simulink model "Imu_sensor_module"  (R2024b)
settings: Solver=VariableStepAuto  StartTime=0.0  StopTime=10  RelTol=1e-3
values from neighbouring files (symbols this model uses):
  bias_acc = [0.01; -0.02; 0.005]    [CalibParams.m]    (also in Calibrated_Data.mat = [-0.00255529989353 0.0383310681174 -0.0164973505603]; ImuCalibrationGui.m = app.BiasAcc)
  bias_gyro = [0.005; -0.005; 0.002]    [CalibParams.m]    (also in Calibrated_Data.mat = [-0.411069831507 0.447881147736 1.44802201926]; ImuCalibrationGui.m = app.BiasGyro)
  scale_acc = [1.01; 0.98; 1.03]    [CalibParams.m]    (also in Calibrated_Data.mat = [2.19824309405 1.51064702678 3.24094019827]; ImuCalibrationGui.m = app.ScaleAcc)
  scale_gyro = [1.00; 1.02; 0.99]    [CalibParams.m]    (also in Calibrated_Data.mat = [1.88477128946 2.18055047165 4.18647933973]; ImuCalibrationGui.m = app.ScaleGyro)
libraries: simulink x6, sharedtransform x1
settings Model: Creator=Admin  LastModifiedBy=Admin
settings DataIOCC: SaveOutput=off  SignalLogging=off  ReturnWorkspaceOutputs=off

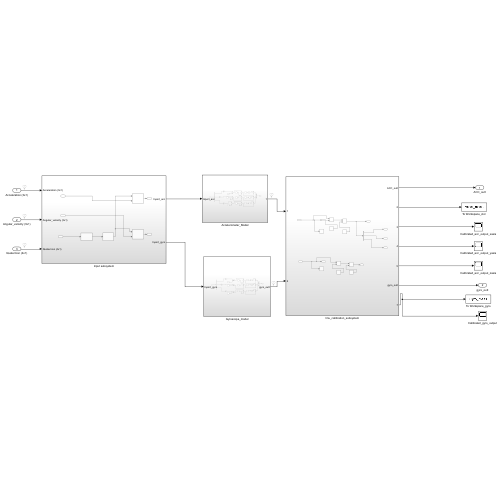
[thumbnail: Simulink's stored preview of the top-level diagram]
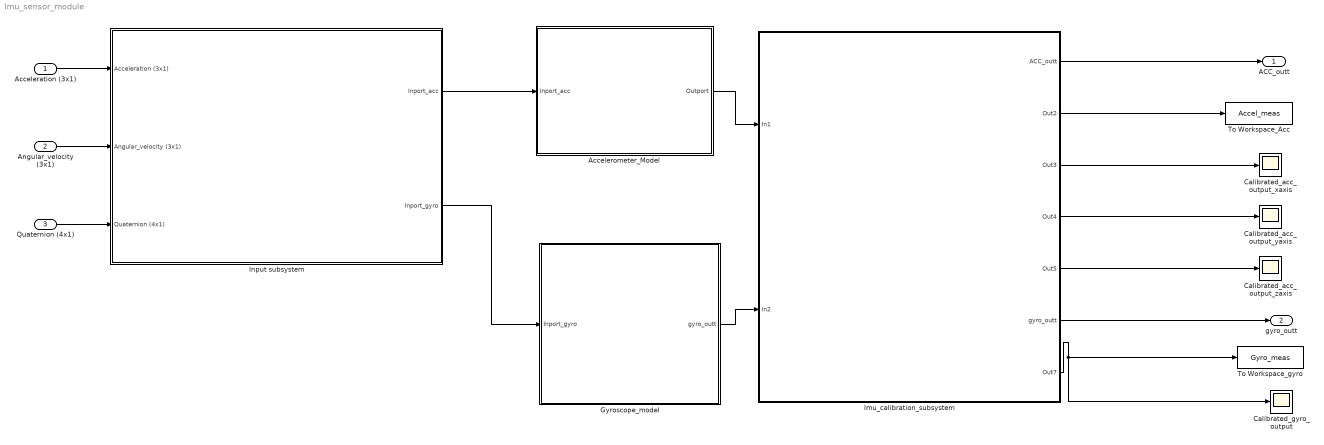
== system Imu_sensor_module ==
  Acceleration (3x1) : Inport  PortDimensions=[3 1]
  Angular_velocity (3x1) : Inport  Port=2  PortDimensions=[3 1]
  Quaternion (4x1) : Inport  Port=3  PortDimensions=[4 1]
  Accelerometer_Model : Subsystem
  Calibrated_acc_output_xaxis : Scope
  Calibrated_acc_output_yaxis : Scope
  Calibrated_acc_output_zaxis : Scope
  Calibrated_gyro_output : Scope
  Gyroscope_model : Subsystem
  Imu_calibration_subsystem : Subsystem
  Input subsystem : Subsystem
  To Workspace_Acc : ToWorkspace  VariableName=Accel_meas  SaveFormat=Structure With Time  SampleTime=-1
  To Workspace_gyro : ToWorkspace  VariableName=Gyro_meas  SaveFormat=Structure With Time  SampleTime=-1
  ACC_outt : Outport
  gyro_outt : Outport  Port=2
  wires:
  Acceleration (3x1)/1 -> Input subsystem/1(Acceleration (3x1))
  Angular_velocity (3x1)/1 -> Input subsystem/2(Angular_velocity (3x1))
  Quaternion (4x1)/1 -> Input subsystem/3(Quaternion (4x1))
  Input subsystem/1(Inport_acc) -> Accelerometer_Model/1(Inport_acc)
  Input subsystem/2(Inport_gyro) -> Gyroscope_model/1(Inport_gyro)
  Imu_calibration_subsystem/7(Out7) -> To Workspace_gyro/1, Calibrated_gyro_output/1
  Accelerometer_Model/1(Outport) -> Imu_calibration_subsystem/1(In1)
  Gyroscope_model/1(gyro_outt) -> Imu_calibration_subsystem/2(In2)
  Imu_calibration_subsystem/1(ACC_outt) -> ACC_outt/1
  Imu_calibration_subsystem/2(Out2) -> To Workspace_Acc/1
  Imu_calibration_subsystem/3(Out3) -> Calibrated_acc_output_xaxis/1
  Imu_calibration_subsystem/4(Out4) -> Calibrated_acc_output_yaxis/1
  Imu_calibration_subsystem/5(Out5) -> Calibrated_acc_output_zaxis/1
  Imu_calibration_subsystem/6(gyro_outt) -> gyro_outt/1

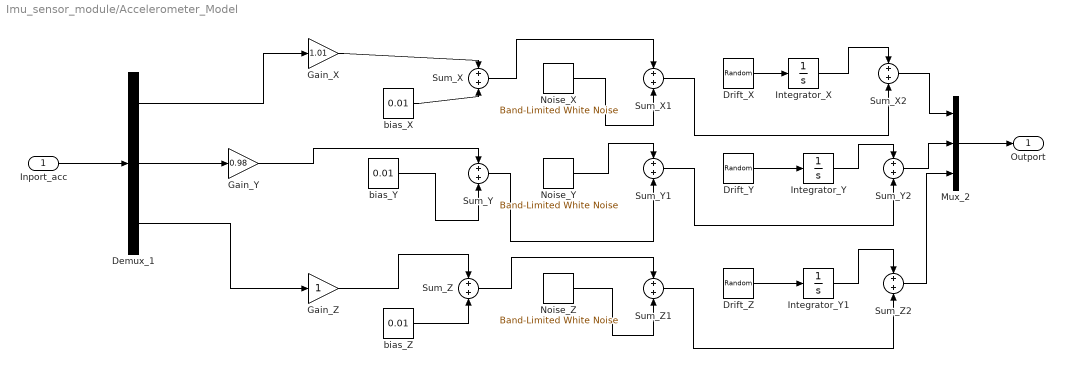
== system Imu_sensor_module/Accelerometer_Model ==
  Inport_acc : Inport  PortDimensions=[3 1]
  Demux_1 : Demux  Outputs=3
  "Drift_X " : RandomNumber  Variance=9e-8  Seed=101  SampleTime=0.01
  Drift_Y : RandomNumber  Variance=7.84e-8  Seed=102  SampleTime=0.01
  Drift_Z : RandomNumber  Variance=6.76e-8  Seed=103  SampleTime=0.01
  Gain_X : Gain  Gain=1.01
  Gain_Y : Gain  Gain=0.98
  Gain_Z : Gain
  "Integrator_X " : Integrator  LimitOutput=on
  Integrator_Y : Integrator  LimitOutput=on
  Integrator_Y1 : Integrator  LimitOutput=on
  Mux_2 : Mux  Inputs=3
      settings: DisplayOption=signals
  "Noise_X " : simulink/Sources/Band-Limited White Noise  Cov=[0.000865]  Ts=0.01  seed=[23341]
  Noise_Y : simulink/Sources/Band-Limited White Noise  Cov=[0.000470]  Ts=0.01  seed=[12345]
  Noise_Z : simulink/Sources/Band-Limited White Noise  Cov=[0.00173]  Ts=0.01  seed=[55000]
  Sum_X : Sum  LockScale=on
  Sum_X1 : Sum  LockScale=on
  Sum_X2 : Sum  LockScale=on
  Sum_Y : Sum  LockScale=on
  Sum_Y1 : Sum  LockScale=on
  Sum_Y2 : Sum  LockScale=on
  Sum_Z : Sum  LockScale=on
  Sum_Z1 : Sum  LockScale=on
  Sum_Z2 : Sum  LockScale=on
  "bias_X " : Constant  Value=0.01
  bias_Y : Constant  Value=0.01
  bias_Z : Constant  Value=0.01
  Outport : Outport
  wires:
  Inport_acc/1 -> Demux_1/1
  Demux_1/1 -> Gain_X/1
  Demux_1/2 -> Gain_Y/1
  Demux_1/3 -> Gain_Z/1
  Gain_X/1 -> Sum_X/1
  "bias_X "/1 -> Sum_X/2
  Gain_Y/1 -> Sum_Y/1
  bias_Y/1 -> Sum_Y/2
  Gain_Z/1 -> Sum_Z/1
  bias_Z/1 -> Sum_Z/2
  Sum_X/1 -> Sum_X1/1
  "Noise_X "/1 -> Sum_X1/2
  Noise_Y/1 -> Sum_Y1/1
  Sum_Y/1 -> Sum_Y1/2
  Sum_Z/1 -> Sum_Z1/1
  Noise_Z/1 -> Sum_Z1/2
  "Drift_X "/1 -> "Integrator_X "/1
  "Integrator_X "/1 -> Sum_X2/1
  Sum_X1/1 -> Sum_X2/2
  Drift_Y/1 -> Integrator_Y/1
  Integrator_Y/1 -> Sum_Y2/1
  Sum_Y1/1 -> Sum_Y2/2
  Drift_Z/1 -> Integrator_Y1/1
  Integrator_Y1/1 -> Sum_Z2/1
  Sum_Z1/1 -> Sum_Z2/2
  Sum_X2/1 -> Mux_2/1
  Sum_Y2/1 -> Mux_2/2
  Sum_Z2/1 -> Mux_2/3
  Mux_2/1 -> Outport/1

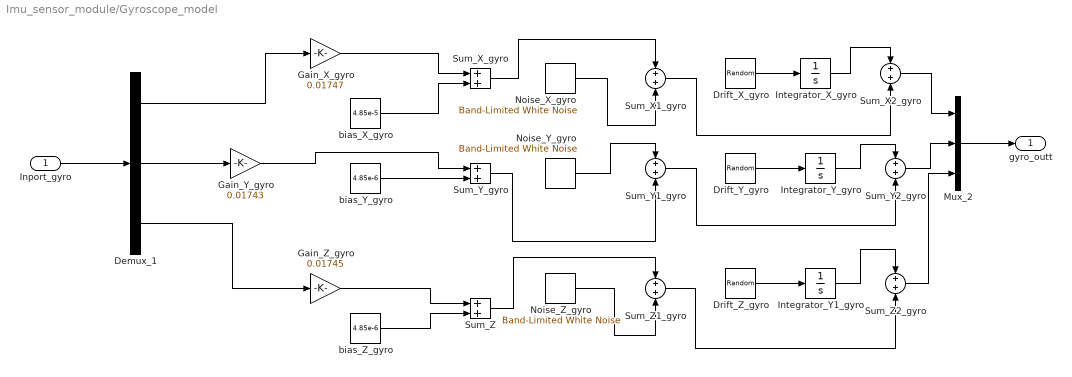
== system Imu_sensor_module/Gyroscope_model ==
  Inport_gyro : Inport  PortDimensions=[3 1]
  " Noise_Z_gyro" : simulink/Sources/Band-Limited White Noise  Cov=[1.25e-4]  Ts=0.01  seed=[55000]
  Demux_1 : Demux  Outputs=3
  "Drift_X_gyro " : RandomNumber  Variance=34.2  Seed=101  SampleTime=0.01
  Drift_Y_gyro : RandomNumber  Variance=34.2  Seed=102  SampleTime=0.01
  Drift_Z_gyro : RandomNumber  Variance=34.2  Seed=103  SampleTime=0.01
  Gain_X_gyro : Gain  Gain=0.01747
  Gain_Y_gyro : Gain  Gain=0.01743
  Gain_Z_gyro : Gain  Gain=0.01745
  "Integrator_X_gyro " : Integrator  LimitOutput=on
  Integrator_Y1_gyro : Integrator  LimitOutput=on
  Integrator_Y_gyro : Integrator  LimitOutput=on
  Mux_2 : Mux  Inputs=3
      settings: DisplayOption=signals
  "Noise_X_gyro " : simulink/Sources/Band-Limited White Noise  Cov=[2.9e-5]  Ts=0.01  seed=[23339]
  Noise_Y_gyro : simulink/Sources/Band-Limited White Noise  Cov=[1.45e-4]  Ts=0.01  seed=[12346]
  Sum_X1_gyro : Sum  LockScale=on
  Sum_X2_gyro : Sum  LockScale=on
  Sum_X_gyro : Sum  LockScale=on
  Sum_Y1_gyro : Sum  LockScale=on
  Sum_Y2_gyro : Sum  LockScale=on
  Sum_Y_gyro : Sum  LockScale=on
  Sum_Z : Sum  LockScale=on
  Sum_Z1_gyro : Sum  LockScale=on
  Sum_Z2_gyro : Sum  LockScale=on
  "bias_X_gyro " : Constant  Value=4.85e-5
  bias_Y_gyro : Constant  Value=4.85e-6
  bias_Z_gyro : Constant  Value=4.85e-6
  gyro_outt : Outport
  wires:
  Sum_Z1_gyro/1 -> Sum_Z2_gyro/2
  "Noise_X_gyro "/1 -> Sum_X1_gyro/2
  Demux_1/3 -> Gain_Z_gyro/1
  " Noise_Z_gyro"/1 -> Sum_Z1_gyro/2
  "Integrator_X_gyro "/1 -> Sum_X2_gyro/1
  bias_Y_gyro/1 -> Sum_Y_gyro/2
  Sum_X2_gyro/1 -> Mux_2/1
  Sum_Z2_gyro/1 -> Mux_2/3
  bias_Z_gyro/1 -> Sum_Z/2
  Sum_X1_gyro/1 -> Sum_X2_gyro/2
  Demux_1/1 -> Gain_X_gyro/1
  Sum_Y2_gyro/1 -> Mux_2/2
  Gain_Z_gyro/1 -> Sum_Z/1
  "Drift_X_gyro "/1 -> "Integrator_X_gyro "/1
  Inport_gyro/1 -> Demux_1/1
  Sum_Z/1 -> Sum_Z1_gyro/1
  Sum_X_gyro/1 -> Sum_X1_gyro/1
  Sum_Y_gyro/1 -> Sum_Y1_gyro/2
  Mux_2/1 -> gyro_outt/1
  Noise_Y_gyro/1 -> Sum_Y1_gyro/1
  Demux_1/2 -> Gain_Y_gyro/1
  Integrator_Y_gyro/1 -> Sum_Y2_gyro/1
  Drift_Z_gyro/1 -> Integrator_Y1_gyro/1
  Sum_Y1_gyro/1 -> Sum_Y2_gyro/2
  Gain_Y_gyro/1 -> Sum_Y_gyro/1
  "bias_X_gyro "/1 -> Sum_X_gyro/2
  Integrator_Y1_gyro/1 -> Sum_Z2_gyro/1
  Gain_X_gyro/1 -> Sum_X_gyro/1
  Drift_Y_gyro/1 -> Integrator_Y_gyro/1

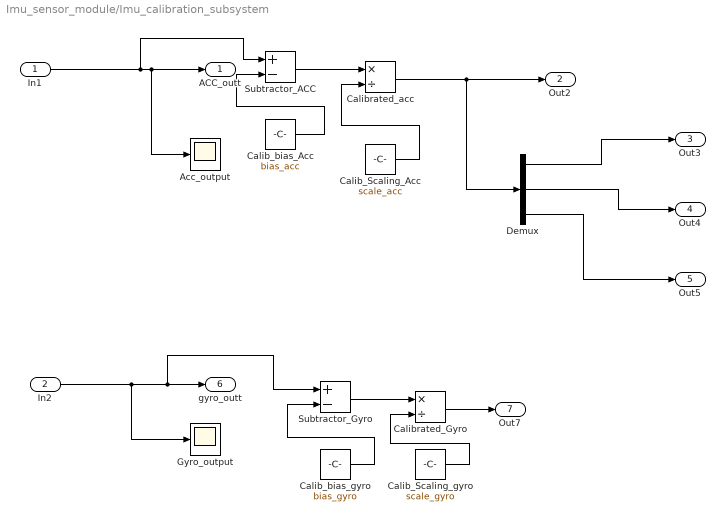
== system Imu_sensor_module/Imu_calibration_subsystem ==
  In1 : Inport
  In2 : Inport  Port=2
  Acc_output : Scope
  Calib_Scaling_Acc : Constant  Value=scale_acc
  Calib_Scaling_gyro : Constant  Value=scale_gyro
  Calib_bias_Acc : Constant  Value=bias_acc
  Calib_bias_gyro : Constant  Value=bias_gyro
  Calibrated_Gyro : Product  Inputs=*/
  Calibrated_acc : Product  Inputs=*/
  Demux : Demux  Outputs=3
  Gyro_output : Scope
  "Subtractor_ACC " : Sum  Inputs=+-
  Subtractor_Gyro : Sum  Inputs=+-
  ACC_outt : Outport
  Out2 : Outport  Port=2
  Out3 : Outport  Port=3
  Out4 : Outport  Port=4
  Out5 : Outport  Port=5
  gyro_outt : Outport  Port=6
  Out7 : Outport  Port=7
  wires:
  "Subtractor_ACC "/1 -> Calibrated_acc/1
  Calib_Scaling_Acc/1 -> Calibrated_acc/2
  Calibrated_Gyro/1 -> Out7/1
  In1/1 -> "Subtractor_ACC "/1, ACC_outt/1, Acc_output/1
  In2/1 -> Gyro_output/1, gyro_outt/1, Subtractor_Gyro/1
  Demux/1 -> Out3/1
  Subtractor_Gyro/1 -> Calibrated_Gyro/1
  Demux/2 -> Out4/1
  Calib_bias_Acc/1 -> "Subtractor_ACC "/2
  Demux/3 -> Out5/1
  Calibrated_acc/1 -> Out2/1, Demux/1
  Calib_bias_gyro/1 -> Subtractor_Gyro/2
  Calib_Scaling_gyro/1 -> Calibrated_Gyro/2

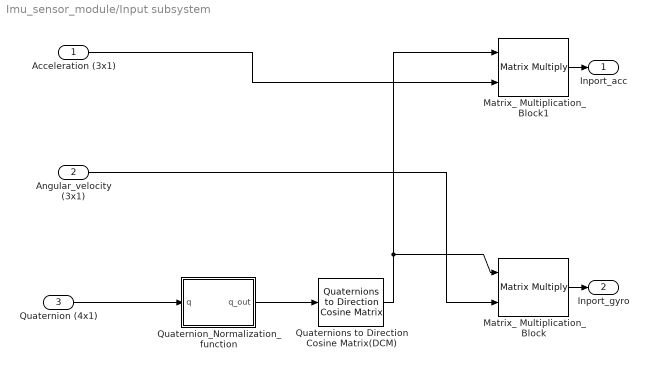
== system Imu_sensor_module/Input subsystem ==
  Acceleration (3x1) : Inport  PortDimensions=[3 1]
  Angular_velocity (3x1) : Inport  Port=2  PortDimensions=[3 1]
  Quaternion (4x1) : Inport  Port=3  PortDimensions=[4 1]
  Matrix_ Multiplication_Block : Product  Multiplication=Matrix(*)
  Matrix_ Multiplication_Block1 : Product  Multiplication=Matrix(*)
  Quaternion_Normalization_function : MATLAB Function  TreatAsAtomicUnit=on
  Quaternions to Direction Cosine Matrix(DCM) : sharedtransform/Quaternions to  Direction Cosine Matrix  aMode=aMode
      settings: LibrarySourceBlock=|
      | aerolibtransform2/Quaternions to
      | Direction Cosine Matrix
  Inport_acc : Outport
  Inport_gyro : Outport  Port=2
  wires:
  Quaternion (4x1)/1 -> Quaternion_Normalization_function/1(q)
  Matrix_ Multiplication_Block1/1 -> Inport_acc/1
  Quaternions to Direction Cosine Matrix(DCM)/1 -> Matrix_ Multiplication_Block/1, Matrix_ Multiplication_Block1/1
  Matrix_ Multiplication_Block/1 -> Inport_gyro/1
  Acceleration (3x1)/1 -> Matrix_ Multiplication_Block1/2
  Angular_velocity (3x1)/1 -> Matrix_ Multiplication_Block/2
  Quaternion_Normalization_function/1(q_out) -> Quaternions to Direction Cosine Matrix(DCM)/1

== matlab function Imu_sensor_module/Input subsystem/Quaternion_Normalization_function ==
  data: q input double size=[4 1]; q_out output
function q_out = safeNormalizeQuaternion(q)

    n = norm(q);
    if n < 1e-6
        q_out = [1; 0; 0; 0];  % Default unit quaternion
    else
        q_out = q / n;
    end
end
